simulink model "gm_sampleModel1541_3_sub"  (R2023a)
settings: Solver=VariableStepAuto  StartTime=0.0  StopTime=10.0  RelTol=1e-3
libraries: simulink x3
settings Model: Creator=user1  LastModifiedBy=user1
settings OptimizationCC: BlockReduction=off  ConditionallyExecuteInputs=off
settings DebuggingCC: InheritedTsInSrcMsg=none

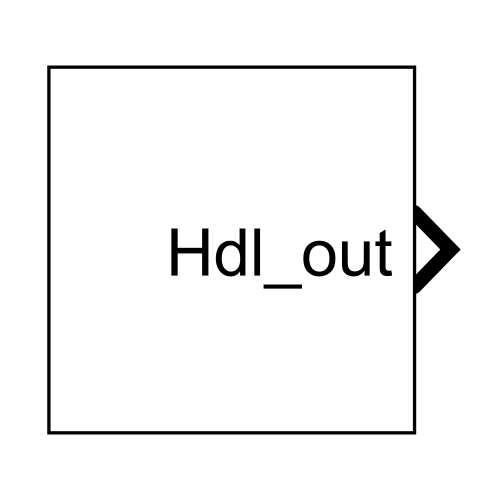
[thumbnail: Simulink's stored preview of the top-level diagram]
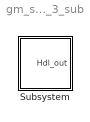
== system gm_sampleModel1541_3_sub ==
  Subsystem : Subsystem

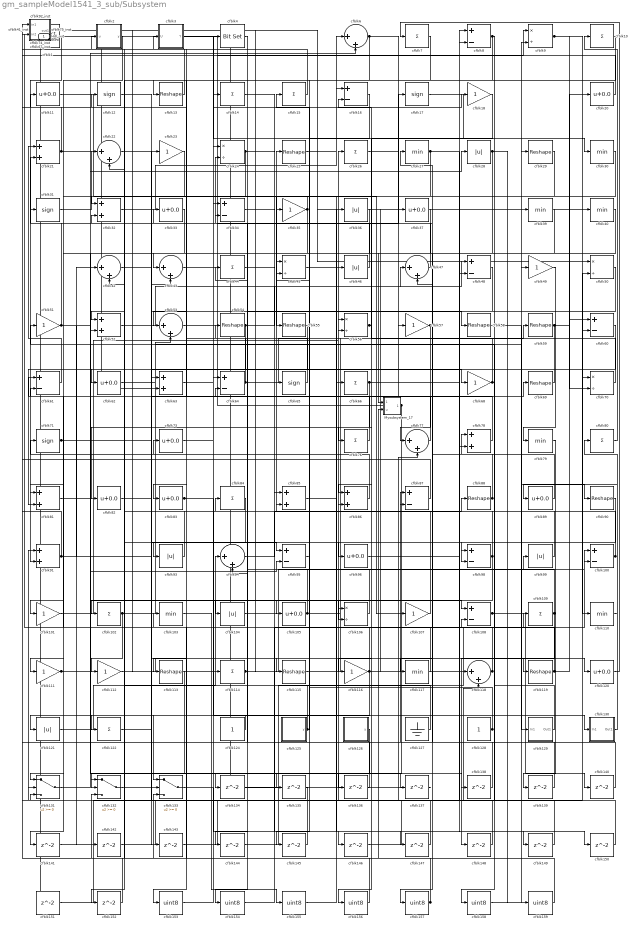
== system gm_sampleModel1541_3_sub/Subsystem ==
  Mysubsystem_17 : Subsystem
  cfblk1 : simulink/Logic and Bit Operations/Detect Decrease  vinit=0.0  OutDataTypeStr=uint8
      settings: LibrarySourceBlock=|
      | hdlsllib/Logic and Bit
      | Operations/Detect
      | Decrease
  cfblk{7,10,14..15,26,44,66,76,80,84,102,109,114,122} (14 alike) : Sum  Inputs=+  OutDataTypeStr=uint8
  cfblk{8,16,34,48,60..61,64,87,95,98,100,108} (12 alike) : Sum  Inputs=+-  OutDataTypeStr=uint8
  cfblk{18,23,35,49,51,57,68,101,107,111..112,116} (12 alike) : Gain  OutDataTypeStr=uint8
  cfblk{27,30,39..40,79,103,110,117} (8 alike) : MinMax  OutDataTypeStr=uint8
  cfblk{28,36,46,93,99,104,121} (7 alike) : Abs  OutDataTypeStr=uint8  SaturateOnIntegerOverflow=off
  cfblk{11,20,33,37,62,73,82..83,89,96,105,120} (12 alike) : Bias  Bias=0.0  SaturateOnIntegerOverflow=off
  cfblk{9,24,45,50,56,70,106} (7 alike) : Product  Inputs=*/  OutDataTypeStr=uint8  RndMeth=Zero  SaturateOnIntegerOverflow=on
  cfblk{13,25,29,54..55,58..59,69,88,90,113,115,119} (13 alike) : Reshape
  cfblk{6,22,42..43,47,53,77,94,118} (9 alike) : Sum  Inputs=|++  OutDataTypeStr=uint8
  cfblk{12,17,31,65,71} (5 alike) : Signum
  cfblk124 : Constant  OutDataTypeStr=uint8  SampleTime=-1
  cfblk125 : Subsystem  mask(Counter Limited){uplimit=double(7), tsamp=double(-1)}
      mask prompts: uplimit "Simulink:masks:UpperLimit_MP"; tsamp "Simulink:masks:SampleTime_MP"
      mask help: Simulink:masks:CounterLimited_MD
      mask init:
      | nbits = double(8);
      | tsamp = double(-1);
      | uplimit = double(7);
  cfblk126 : Subsystem  mask(Counter Free-Running){NumBits=double(16), tsamp=double(-1)}
      mask prompts: NumBits "Simulink:masks:NumberOfBits_MP"; tsamp "Simulink:masks:SampleTime_MP"
      mask help: Simulink:masks:CounterFreeRunning_MD
  cfblk127 : Ground
  cfblk128 : Constant  OutDataTypeStr=uint8  SampleTime=-1
  cfblk129 : Subsystem
  cfblk130 : Subsystem
  cfblk131 : Switch  OutDataTypeStr=uint8  SaturateOnIntegerOverflow=off  InputSameDT=off
  cfblk132 : Switch  OutDataTypeStr=uint8  SaturateOnIntegerOverflow=off  InputSameDT=off
  cfblk133 : Switch  OutDataTypeStr=uint8  SaturateOnIntegerOverflow=off  InputSameDT=off
  cfblk{134..152} (19 alike) : Delay  SampleTime=1
  cfblk{153..159} (7 alike) : DataTypeConversion  OutDataTypeStr=uint8  SaturateOnIntegerOverflow=off  RndMeth=Floor
  cfblk2 : Subsystem  mask(Compare To Zero){relop=<=, OutDataTypeStr=uint8, ZeroCross=on}
      mask prompts: relop "Simulink:masks:Operator_MP"; OutDataTypeStr "Simulink:masks:OutputDataType_MP"; ZeroCross "Simulink:masks:EnableZerocrossingDetection_MP"
      mask help: Simulink:masks:CompareToZero_MD
      mask init:
      | OutDataTypeStr = 'uint8';
      | ZeroCross = 'on';
      | blkName = 'sampleModel1541_3_sub/Subsystem/cfblk2';
      | relop = '<=';
      | setValue = 'fixdt(0, 8)';
      mask TypeOptions relop: == | ~= | < | <= | >= | >
      mask TypeOptions OutDataTypeStr: Simulink:masks:uint8 | Simulink:masks:boolean
      mask Callback ZeroCross: sl('zeroCrossEnable', gcbh);
      mask Display: disp([relop,' 0'])
  cfblk{21,32,52,63,78,81,85..86,91} (9 alike) : Sum  OutDataTypeStr=uint8
  cfblk3 : Subsystem  mask(Detect Fall Negative){vinit=double(0), InputProcessing=Elements as channels (sample based), OutDataTypeStr=uint8}
      mask prompts: vinit "Simulink:masks:InitialCondition_MP"; InputProcessing "Simulink:masks:InputProcessing_MP"; OutDataTypeStr "Simulink:masks:OutputDataType_MP"
      mask help: Simulink:masks:DetectFallNegative_MD
      mask init:
      | InputProcessing = 'Elements as channels (sample based)';
      | OutDataTypeStr = 'uint8';
      | vinit = double(0);
      mask TypeOptions InputProcessing: Simulink:masks:ColumnsAsChannelsFrameBased | Simulink:masks:ElementsAsChannelsSampleBased
      mask TypeOptions OutDataTypeStr: Simulink:masks:uint8 | Simulink:masks:boolean
      mask Display: fprintf('U < 0\n&  NOT\nU/z < 0')
  cfblk38_inst : Subsystem
  cfblk4 : simulink/Logic and Bit Operations/Bit Set  iBit=0
      settings: LibrarySourceBlock=|
      | hdlsllib/Logic and Bit
      | Operations/Bit Set
  cfblk41_inst : Subsystem
  cfblk67_inst : Subsystem
  cfblk74_inst : Subsystem
  cfblk75_inst : Subsystem
  cfblk92_inst : Subsystem
  Hdl_out : Outport  OutDataTypeStr=uint8  SampleTime=1
  wires:
  Mysubsystem_17/1(Out1) -> cfblk134/1, Hdl_out/1
  cfblk1/1 -> cfblk91/2
  cfblk10/1 -> cfblk13/1
  cfblk100/1 -> cfblk42/2, cfblk26/1
  cfblk101/1 -> cfblk56/1
  cfblk102/1 -> cfblk53/2, cfblk112/1
  cfblk103/1 -> cfblk155/1
  cfblk104/1 -> cfblk99/1
  cfblk105/1 -> cfblk32/2, cfblk100/1
  cfblk106/1 -> cfblk71/1
  cfblk107/1 -> cfblk25/1
  cfblk108/1 -> cfblk49/1, cfblk140/1
  cfblk109/1 -> cfblk73/1, cfblk148/1
  cfblk11/1 -> cfblk55/1
  cfblk110/1 -> cfblk89/1
  cfblk111/1 -> cfblk95/2, cfblk6/2
  cfblk112/1 -> cfblk120/1
  cfblk113/1 -> cfblk132/2
  cfblk114/1 -> cfblk46/1, cfblk108/2
  cfblk115/1 -> cfblk59/1
  cfblk116/1 -> cfblk37/1, cfblk133/1, cfblk45/1
  cfblk117/1 -> cfblk75_inst/2(in2)
  cfblk118/1 -> cfblk61/2, cfblk15/1
  cfblk119/1 -> cfblk94/2, cfblk20/1
  cfblk12/1 -> cfblk115/1
  cfblk120/1 -> cfblk7/1
  cfblk121/1 -> cfblk94/1
  cfblk122/1 -> cfblk23/1
  cfblk124/1 -> cfblk121/1
  cfblk125/1(y) -> cfblk45/2, cfblk84/1
  cfblk126/1(y) -> cfblk132/1
  cfblk127/1 -> cfblk22/2
  cfblk128/1 -> cfblk85/2, cfblk56/2
  cfblk129/1(Out1) -> cfblk51/1
  cfblk13/1 -> cfblk75_inst/1(in1)
  cfblk130/1(Out1) -> cfblk80/1
  cfblk131/1 -> cfblk28/1
  cfblk132/1 -> cfblk69/1
  cfblk133/1 -> cfblk146/1
  cfblk134/1 -> cfblk50/2
  cfblk135/1 -> cfblk131/3
  cfblk136/1 -> cfblk64/2
  cfblk137/1 -> cfblk1/1
  cfblk138/1 -> cfblk47/2
  cfblk139/1 -> cfblk87/1
  cfblk14/1 -> cfblk137/1
  cfblk140/1 -> cfblk38_inst/2(in2)
  cfblk141/1 -> cfblk43/2
  cfblk142/1 -> cfblk70/1
  cfblk143/1 -> cfblk77/2
  cfblk144/1 -> cfblk100/2
  cfblk145/1 -> cfblk91/1
  cfblk146/1 -> cfblk8/2
  cfblk147/1 -> cfblk74_inst/1(in1)
  cfblk148/1 -> cfblk86/2
  cfblk149/1 -> cfblk131/2
  cfblk15/1 -> cfblk74_inst/2(in2)
  cfblk150/1 -> cfblk78/1
  cfblk151/1 -> cfblk118/2
  cfblk152/1 -> cfblk41_inst/2(in2)
  cfblk153/1 -> cfblk4/1
  cfblk154/1 -> cfblk109/1
  cfblk155/1 -> cfblk36/1
  cfblk156/1 -> cfblk103/1
  cfblk157/1 -> cfblk133/3, cfblk132/3, cfblk12/1
  cfblk158/1 -> cfblk39/1
  cfblk159/1 -> Mysubsystem_17/2(u)
  cfblk16/1 -> cfblk145/1
  cfblk17/1 -> cfblk110/1
  cfblk18/1 -> cfblk96/1
  cfblk2/1(y) -> cfblk111/1
  cfblk20/1 -> cfblk92_inst/2(in2)
  cfblk21/1 -> cfblk67_inst/1(in1), cfblk107/1, cfblk66/1
  cfblk22/1 -> cfblk68/1
  cfblk23/1 -> cfblk52/1
  cfblk24/1 -> cfblk113/1, cfblk136/1
  cfblk25/1 -> cfblk16/1
  cfblk26/1 -> cfblk57/1
  cfblk27/1 -> cfblk119/1, cfblk116/1
  cfblk28/1 -> cfblk78/2, cfblk159/1, Mysubsystem_17/1(In1)
  cfblk29/1 -> cfblk101/1
  cfblk3/1(Y) -> cfblk30/1
  cfblk30/1 -> cfblk156/1
  cfblk31/1 -> cfblk22/1
  cfblk32/1 -> cfblk6/1
  cfblk33/1 -> cfblk81/1
  cfblk34/1 -> cfblk85/1
  cfblk35/1 -> cfblk52/2, cfblk32/1, cfblk141/1
  cfblk36/1 -> cfblk43/1
  cfblk37/1 -> cfblk86/1
  cfblk38_inst/1(out1) -> cfblk118/1
  cfblk39/1 -> cfblk157/1
  cfblk4/1 -> cfblk154/1
  cfblk40/1 -> cfblk104/1
  cfblk41_inst/1(out1) -> cfblk38_inst/1(in1)
  cfblk42/1 -> cfblk58/1
  cfblk43/1 -> cfblk9/1
  cfblk44/1 -> cfblk150/1
  cfblk45/1 -> cfblk147/1
  cfblk46/1 -> cfblk24/2
  cfblk47/1 -> cfblk34/2
  cfblk48/1 -> cfblk144/1
  cfblk49/1 -> cfblk79/1
  cfblk50/1 -> cfblk105/1
  cfblk51/1 -> cfblk21/2, cfblk133/2, cfblk142/1
  cfblk52/1 -> cfblk47/1
  cfblk53/1 -> cfblk17/1
  cfblk54/1 -> cfblk48/1, cfblk153/1
  cfblk55/1 -> cfblk131/1
  cfblk56/1 -> cfblk106/2, cfblk76/1
  cfblk57/1 -> cfblk77/1, cfblk117/1
  cfblk58/1 -> cfblk90/1
  cfblk59/1 -> cfblk81/2, cfblk60/1
  cfblk6/1 -> cfblk53/1, cfblk129/1(In1)
  cfblk60/1 -> cfblk135/1
  cfblk61/1 -> cfblk21/1
  cfblk62/1 -> cfblk29/1
  cfblk63/1 -> cfblk14/1
  cfblk64/1 -> cfblk11/1, cfblk9/2
  cfblk65/1 -> cfblk34/1
  cfblk66/1 -> cfblk82/1, cfblk48/2
  cfblk67_inst/1(out1) -> cfblk63/2
  cfblk68/1 -> cfblk98/2, cfblk16/2, cfblk158/1
  cfblk69/1 -> cfblk62/1
  cfblk7/1 -> cfblk35/1
  cfblk70/1 -> cfblk8/1
  cfblk71/1 -> cfblk108/1, cfblk138/1
  cfblk73/1 -> cfblk24/1
  cfblk74_inst/1(out1) -> cfblk50/1
  cfblk75_inst/1(out1) -> cfblk151/1, cfblk40/1
  cfblk76/1 -> cfblk63/1
  cfblk77/1 -> cfblk64/1
  cfblk78/1 -> cfblk3/1(U)
  cfblk79/1 -> cfblk139/1
  cfblk8/1 -> cfblk98/1, cfblk83/1, cfblk102/1
  cfblk80/1 -> cfblk10/1
  cfblk81/1 -> cfblk106/1
  cfblk82/1 -> cfblk143/1
  cfblk83/1 -> cfblk18/1, cfblk130/1(In1)
  cfblk84/1 -> cfblk93/1
  cfblk85/1 -> cfblk87/2
  cfblk86/1 -> cfblk54/1
  cfblk87/1 -> cfblk92_inst/1(in1)
  cfblk88/1 -> cfblk61/1, cfblk33/1
  cfblk89/1 -> cfblk31/1
  cfblk9/1 -> cfblk60/2, cfblk70/2
  cfblk90/1 -> cfblk152/1
  cfblk91/1 -> cfblk95/1, cfblk42/1, cfblk41_inst/1(in1)
  cfblk92_inst/1(out1) -> cfblk67_inst/2(in2), cfblk114/1
  cfblk93/1 -> cfblk2/1(u)
  cfblk94/1 -> cfblk88/1
  cfblk95/1 -> cfblk65/1
  cfblk96/1 -> cfblk149/1
  cfblk98/1 -> cfblk122/1, cfblk27/1
  cfblk99/1 -> cfblk44/1

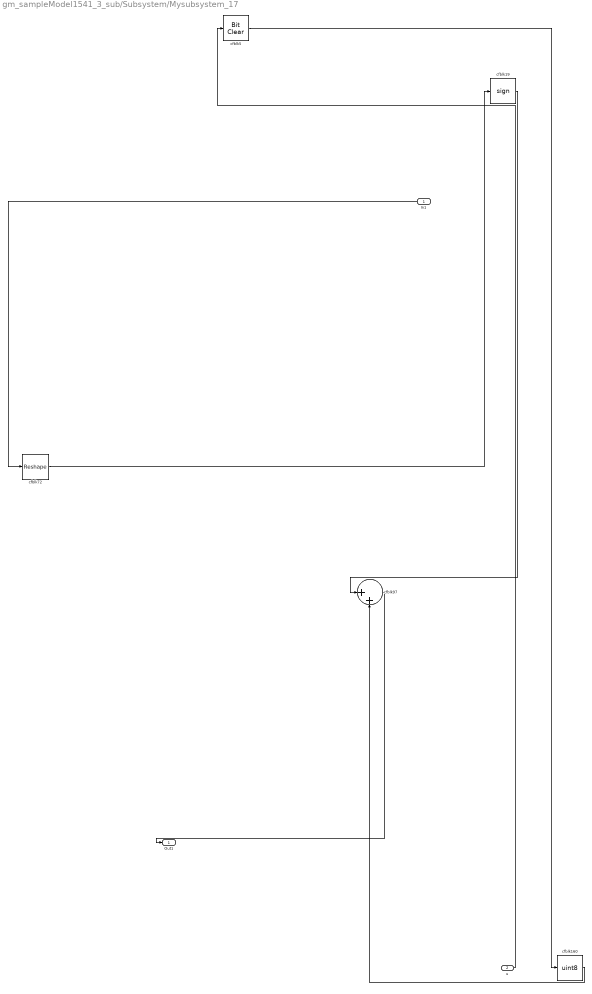
== system gm_sampleModel1541_3_sub/Subsystem/Mysubsystem_17 ==
  In1 : Inport  OutDataTypeStr=uint8  PortDimensions=1  SampleTime=1
  u : Inport  Port=2  OutDataTypeStr=uint8  PortDimensions=1  SampleTime=1
  cfblk160 : DataTypeConversion  OutDataTypeStr=uint8  SaturateOnIntegerOverflow=off  RndMeth=Floor
  cfblk19 : Signum
  cfblk5 : simulink/Logic and Bit Operations/Bit Clear  iBit=0
      settings: LibrarySourceBlock=|
      | hdlsllib/Logic and Bit
      | Operations/Bit Clear
  cfblk72 : Reshape
  cfblk97 : Sum  Inputs=|++
  Out1 : Outport  SampleTime=1
  wires:
  In1/1 -> cfblk72/1
  u/1 -> cfblk5/1
  cfblk160/1 -> cfblk97/2
  cfblk19/1 -> cfblk97/1
  cfblk5/1 -> cfblk160/1
  cfblk72/1 -> cfblk19/1
  cfblk97/1 -> Out1/1

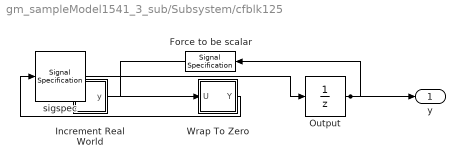
== system gm_sampleModel1541_3_sub/Subsystem/cfblk125 ==
  Force to be scalar : SignalSpecification  DisableCoverage=on  Dimensions=1
  Increment Real World : Subsystem  mask(Real World Value Increment){}
      mask help: Simulink:masks:RealWorldValueIncrement_MD
      mask Display: disp('V++')
  Output : UnitDelay  InitialCondition=0.0  SampleTime=tsamp  HasFrameUpgradeWarning=on
  Wrap To Zero : Subsystem  mask(Wrap To Zero){Threshold=double(7)}
      mask prompts: Threshold "Simulink:masks:Threshold_MP"
      mask help: Simulink:masks:WrapToZero_MD
  sigspec : SignalSpecification  OutDataTypeStr=uint8  Dimensions=1
  y : Outport  SampleTime=1
  wires:
  Force to be scalar/1 -> Increment Real World/1(u)
  Increment Real World/1(y) -> Wrap To Zero/1(U)
  Output/1 -> Force to be scalar/1, y/1
  Wrap To Zero/1(Y) -> sigspec/1
  sigspec/1 -> Output/1

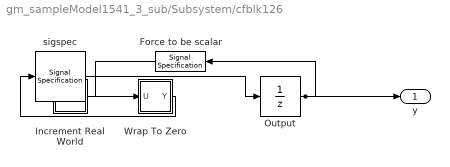
== system gm_sampleModel1541_3_sub/Subsystem/cfblk126 ==
  Force to be scalar : SignalSpecification  DisableCoverage=on  Dimensions=1
  Increment Real World : Subsystem  mask(Real World Value Increment){}
      mask help: Simulink:masks:RealWorldValueIncrement_MD
      mask Display: disp('V++')
  Output : UnitDelay  InitialCondition=0.0  SampleTime=tsamp  HasFrameUpgradeWarning=on
  Wrap To Zero : Subsystem  mask(Wrap To Zero){Threshold=double(65535)}
      mask prompts: Threshold "Simulink:masks:Threshold_MP"
      mask help: Simulink:masks:WrapToZero_MD
  sigspec : SignalSpecification  OutDataTypeStr=uint16  Dimensions=1
  y : Outport  SampleTime=1
  wires:
  Force to be scalar/1 -> Increment Real World/1(u)
  Increment Real World/1(y) -> Wrap To Zero/1(U)
  Output/1 -> Force to be scalar/1, y/1
  Wrap To Zero/1(Y) -> sigspec/1
  sigspec/1 -> Output/1

== system gm_sampleModel1541_3_sub/Subsystem/cfblk129 ==
  In1 : Inport  OutDataTypeStr=uint8  PortDimensions=1  SampleTime=1
  Out1 : Outport  SampleTime=1
  wires:
  In1/1 -> Out1/1

== system gm_sampleModel1541_3_sub/Subsystem/cfblk130 ==
  In1 : Inport  OutDataTypeStr=uint8  PortDimensions=1  SampleTime=1
  Out1 : Outport  SampleTime=1
  wires:
  In1/1 -> Out1/1

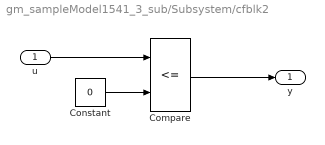
== system gm_sampleModel1541_3_sub/Subsystem/cfblk2 ==
  u : Inport  OutDataTypeStr=uint8  SampleTime=1
  Compare : RelationalOperator  Operator=<=  OutDataTypeStr=fixdt(0, 8)
  Constant : Constant  DisableCoverage=on  Value=0  OutDataTypeStr=Inherit: Inherit via back propagation  SampleTime=-1  PreserveConstantTs=on
  y : Outport  SampleTime=1
  wires:
  u/1 -> Compare/1
  Compare/1 -> y/1
  Constant/1 -> Compare/2

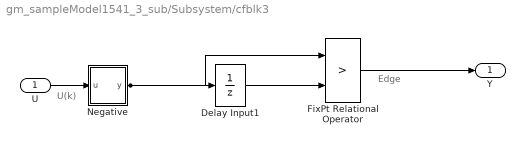
== system gm_sampleModel1541_3_sub/Subsystem/cfblk3 ==
  note: U(k)
  note: Edge
  U : Inport  OutDataTypeStr=uint8  SampleTime=1
  Delay Input1 : UnitDelay  Description=Store in Global RAM  DisableCoverage=on  InitialCondition=vinit  SampleTime=-1  HasFrameUpgradeWarning=on
  FixPt Relational Operator : RelationalOperator  Operator=>  OutDataTypeStr=fixdt(0, 8)  ZeroCross=off  InputSameDT=off
  Negative : Subsystem  mask(Compare To Zero){relop=<, OutDataTypeStr=boolean, ZeroCross=off}
      mask prompts: relop "Simulink:masks:Operator_MP"; OutDataTypeStr "Simulink:masks:OutputDataType_MP"; ZeroCross "Simulink:masks:EnableZerocrossingDetection_MP"
      mask help: Simulink:masks:CompareToZero_MD
      mask init:
      | OutDataTypeStr = 'boolean';
      | ZeroCross = 'off';
      | blkName = 'sampleModel1541_3_sub/Subsystem/cfblk3/Negative';
      | relop = '<';
      | setValue = 'boolean';
      mask TypeOptions relop: == | ~= | < | <= | >= | >
      mask TypeOptions OutDataTypeStr: Simulink:masks:uint8 | Simulink:masks:boolean
      mask Callback ZeroCross: sl('zeroCrossEnable', gcbh);
      mask Display: disp([relop,' 0'])
  Y : Outport  SampleTime=1
  wires:
  U/1 -> Negative/1(u)
  Delay Input1/1 -> FixPt Relational Operator/2
  FixPt Relational Operator/1 -> Y/1
  Negative/1(y) -> FixPt Relational Operator/1, Delay Input1/1

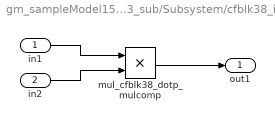
== system gm_sampleModel1541_3_sub/Subsystem/cfblk38_inst ==
  in1 : Inport  OutDataTypeStr=uint8  SampleTime=1
  in2 : Inport  Port=2  OutDataTypeStr=uint8  SampleTime=1
  mul_cfblk38_dotp_mulcomp : Product  Inputs=**  OutDataTypeStr=uint8  SampleTime=1
  out1 : Outport  OutDataTypeStr=uint8  SampleTime=1
  wires:
  in1/1 -> mul_cfblk38_dotp_mulcomp/1
  in2/1 -> mul_cfblk38_dotp_mulcomp/2
  mul_cfblk38_dotp_mulcomp/1 -> out1/1

== system gm_sampleModel1541_3_sub/Subsystem/cfblk41_inst ==
  in1 : Inport  OutDataTypeStr=uint8  SampleTime=1
  in2 : Inport  Port=2  OutDataTypeStr=uint8  SampleTime=1
  mul_cfblk41_dotp_mulcomp : Product  Inputs=**  OutDataTypeStr=uint8  SampleTime=1
  out1 : Outport  OutDataTypeStr=uint8  SampleTime=1
  wires:
  in1/1 -> mul_cfblk41_dotp_mulcomp/1
  in2/1 -> mul_cfblk41_dotp_mulcomp/2
  mul_cfblk41_dotp_mulcomp/1 -> out1/1

== system gm_sampleModel1541_3_sub/Subsystem/cfblk67_inst ==
  in1 : Inport  OutDataTypeStr=uint8  SampleTime=1
  in2 : Inport  Port=2  OutDataTypeStr=uint8  SampleTime=1
  mul_cfblk67_dotp_mulcomp : Product  Inputs=**  OutDataTypeStr=uint8  SampleTime=1
  out1 : Outport  OutDataTypeStr=uint8  SampleTime=1
  wires:
  in1/1 -> mul_cfblk67_dotp_mulcomp/1
  in2/1 -> mul_cfblk67_dotp_mulcomp/2
  mul_cfblk67_dotp_mulcomp/1 -> out1/1

== system gm_sampleModel1541_3_sub/Subsystem/cfblk74_inst ==
  in1 : Inport  OutDataTypeStr=uint8  SampleTime=1
  in2 : Inport  Port=2  OutDataTypeStr=uint8  SampleTime=1
  mul_cfblk74_dotp_mulcomp : Product  Inputs=**  OutDataTypeStr=uint8  SampleTime=1
  out1 : Outport  OutDataTypeStr=uint8  SampleTime=1
  wires:
  in1/1 -> mul_cfblk74_dotp_mulcomp/1
  in2/1 -> mul_cfblk74_dotp_mulcomp/2
  mul_cfblk74_dotp_mulcomp/1 -> out1/1

== system gm_sampleModel1541_3_sub/Subsystem/cfblk75_inst ==
  in1 : Inport  OutDataTypeStr=uint8  SampleTime=1
  in2 : Inport  Port=2  OutDataTypeStr=uint8  SampleTime=1
  mul_cfblk75_dotp_mulcomp : Product  Inputs=**  OutDataTypeStr=uint8  SampleTime=1
  out1 : Outport  OutDataTypeStr=uint8  SampleTime=1
  wires:
  in1/1 -> mul_cfblk75_dotp_mulcomp/1
  in2/1 -> mul_cfblk75_dotp_mulcomp/2
  mul_cfblk75_dotp_mulcomp/1 -> out1/1

== system gm_sampleModel1541_3_sub/Subsystem/cfblk92_inst ==
  in1 : Inport  OutDataTypeStr=uint8  SampleTime=1
  in2 : Inport  Port=2  OutDataTypeStr=uint8  SampleTime=1
  mul_cfblk92_dotp_mulcomp : Product  Inputs=**  OutDataTypeStr=uint8  SampleTime=1
  out1 : Outport  OutDataTypeStr=uint8  SampleTime=1
  wires:
  in1/1 -> mul_cfblk92_dotp_mulcomp/1
  in2/1 -> mul_cfblk92_dotp_mulcomp/2
  mul_cfblk92_dotp_mulcomp/1 -> out1/1

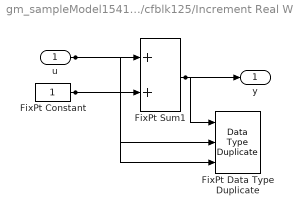
== system gm_sampleModel1541_3_sub/Subsystem/cfblk125/Increment Real World ==
  u : Inport  OutDataTypeStr=uint8  SampleTime=1
  FixPt Constant : Constant  DisableCoverage=on  OutDataTypeStr=Inherit: Inherit via back propagation  SampleTime=-1
  FixPt Data Type Duplicate : DataTypeDuplicate  DisableCoverage=on  NumInputPorts=3
  FixPt Sum1 : Sum  InputSameDT=on  OutDataTypeStr=Inherit: Inherit via back propagation  LockScale=on
  y : Outport  SampleTime=1
  wires:
  u/1 -> FixPt Sum1/1, FixPt Data Type Duplicate/2
  FixPt Constant/1 -> FixPt Sum1/2, FixPt Data Type Duplicate/3
  FixPt Sum1/1 -> FixPt Data Type Duplicate/1, y/1

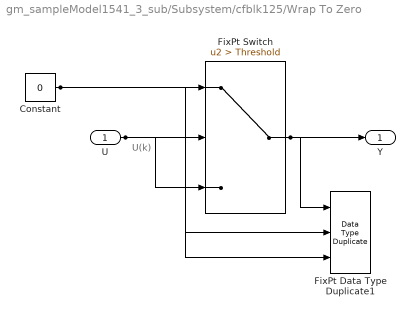
== system gm_sampleModel1541_3_sub/Subsystem/cfblk125/Wrap To Zero ==
  note: U(k)
  U : Inport  OutDataTypeStr=uint8  SampleTime=1
  Constant : Constant  DisableCoverage=on  Value=0  OutDataTypeStr=Inherit: Inherit via back propagation  SampleTime=-1
  FixPt Data Type Duplicate1 : DataTypeDuplicate  DisableCoverage=on  NumInputPorts=3
  FixPt Switch : Switch  Criteria=u2 > Threshold  Threshold=Threshold  OutDataTypeStr=Inherit: Inherit via back propagation  ZeroCross=off  SaturateOnIntegerOverflow=off  InputSameDT=off
  Y : Outport  SampleTime=1
  wires:
  U/1 -> FixPt Switch/3, FixPt Switch/2, FixPt Data Type Duplicate1/2
  Constant/1 -> FixPt Switch/1, FixPt Data Type Duplicate1/3
  FixPt Switch/1 -> FixPt Data Type Duplicate1/1, Y/1

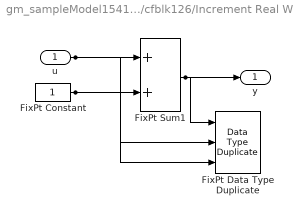
== system gm_sampleModel1541_3_sub/Subsystem/cfblk126/Increment Real World ==
  u : Inport  OutDataTypeStr=uint16  SampleTime=1
  FixPt Constant : Constant  DisableCoverage=on  OutDataTypeStr=Inherit: Inherit via back propagation  SampleTime=-1
  FixPt Data Type Duplicate : DataTypeDuplicate  DisableCoverage=on  NumInputPorts=3
  FixPt Sum1 : Sum  InputSameDT=on  OutDataTypeStr=Inherit: Inherit via back propagation  LockScale=on
  y : Outport  SampleTime=1
  wires:
  u/1 -> FixPt Sum1/1, FixPt Data Type Duplicate/2
  FixPt Constant/1 -> FixPt Sum1/2, FixPt Data Type Duplicate/3
  FixPt Sum1/1 -> FixPt Data Type Duplicate/1, y/1

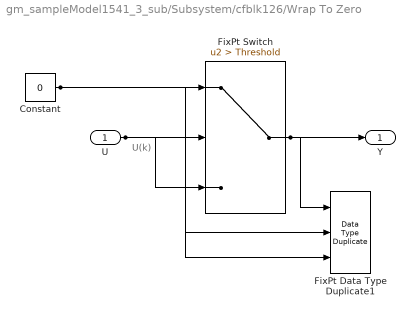
== system gm_sampleModel1541_3_sub/Subsystem/cfblk126/Wrap To Zero ==
  note: U(k)
  U : Inport  OutDataTypeStr=uint16  SampleTime=1
  Constant : Constant  DisableCoverage=on  Value=0  OutDataTypeStr=Inherit: Inherit via back propagation  SampleTime=-1
  FixPt Data Type Duplicate1 : DataTypeDuplicate  DisableCoverage=on  NumInputPorts=3
  FixPt Switch : Switch  Criteria=u2 > Threshold  Threshold=Threshold  OutDataTypeStr=Inherit: Inherit via back propagation  ZeroCross=off  SaturateOnIntegerOverflow=off  InputSameDT=off
  Y : Outport  SampleTime=1
  wires:
  U/1 -> FixPt Switch/3, FixPt Switch/2, FixPt Data Type Duplicate1/2
  Constant/1 -> FixPt Switch/1, FixPt Data Type Duplicate1/3
  FixPt Switch/1 -> FixPt Data Type Duplicate1/1, Y/1

== system gm_sampleModel1541_3_sub/Subsystem/cfblk3/Negative ==
  u : Inport  OutDataTypeStr=uint8  SampleTime=1
  Compare : RelationalOperator  Operator=<  OutDataTypeStr=boolean  ZeroCross=off
  Constant : Constant  DisableCoverage=on  Value=0  OutDataTypeStr=Inherit: Inherit via back propagation  SampleTime=-1  PreserveConstantTs=on
  y : Outport  SampleTime=1
  wires:
  u/1 -> Compare/1
  Compare/1 -> y/1
  Constant/1 -> Compare/2
